simulink model "fig82_SistemaFiltroSintonizado"  (R2021a)
settings: Solver=VariableStepAuto  StartTime=0.0  StopTime=5/60  FixedStep=1/(60*512)  MaxStep=0.1e-3  RelTol=1e-3  EnableMultiTasking=on
InitFcn:
  | Ts = 1/(60*512);
undefined symbols (not defined in the file): D11, Delta
libraries: spsCurrentMeasurementLib x27, spsVoltageMeasurementLib x23, spsSeriesRLCBranchLib x7, spsFourierLib x6, spsThreePhaseTransformerTwoWindingsLib x4, spsUniversalBridgeLib x3, spsTHDLib x3, spsParallelRLCBranchLib x2, spsThreePhaseSeriesRLCBranchLib x1, spsGroundLib x1, spsACCurrentSourceLib x1, spsImpedanceMeasurementLib x1
settings Model: Creator=ajust  LastModifiedBy=ajust
settings SolverCC: AlgebraicLoopSolver=TrustRegion
settings DataIOCC: ReturnWorkspaceOutputs=off
settings OptimizationCC: LifeSpan=inf
settings DebuggingCC: AllowSymbolicDim=off  SFUnexpectedBacktrackingDiag=warning  SFNoUnconditionalDefaultTransitionDiag=warning  SFExecutionAtInitializationDiag=none  SFMachineParentedDataDiag=warning  ArithmeticOperatorsInVariantConditions=warning
settings ModelReferenceCC: PropagateSignalLabelsOutOfModel=off
settings SFSimCC: SimUseLocalCustomCode=off  CustomCodeUndefinedFunction=UseInterfaceOnly
settings RTWCC: RTWUseLocalCustomCode=off
settings CodeAppCC: StateflowObjectComments=on
settings GRTTargetCC: TargetLangStandard=C89/C90 (ANSI)
settings ConfigComp: CovMetricSettings=dw  CovSaveCumulativeToWorkspaceVar=on  CovSaveSingleToWorkspaceVar=on  CovExternalEMLEnable=off
settings SimscapeCC: SimscapeNormalizeSystem=off

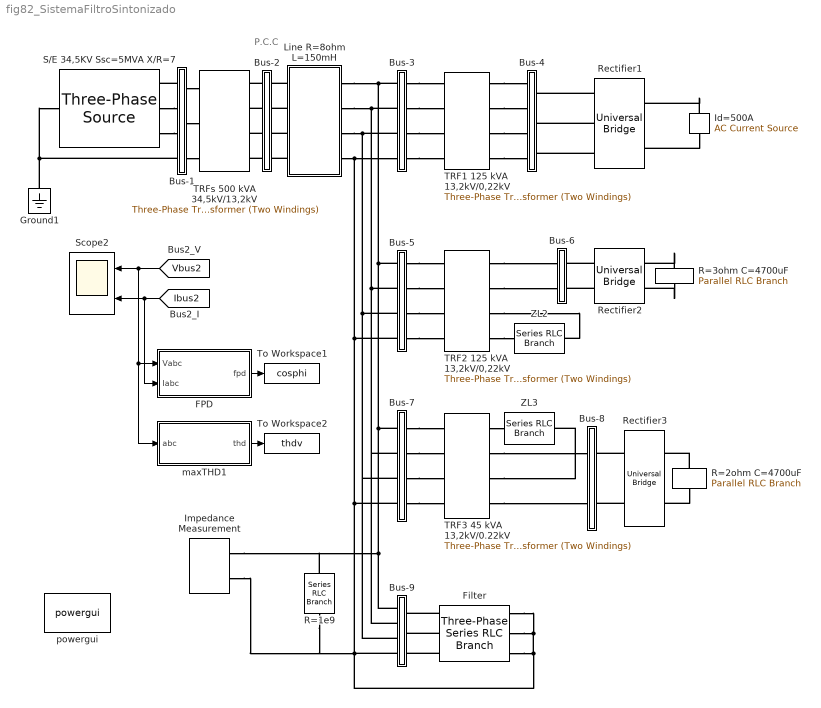
== system fig82_SistemaFiltroSintonizado ==
  note: P.C.C
  Bus-1 : Subsystem
  Bus-2 : Subsystem
  Bus-3 : Subsystem
  Bus-4 : Subsystem
  Bus-5 : Subsystem
  Bus-6 : Subsystem
  Bus-7 : Subsystem
  Bus-8 : Subsystem
  Bus-9 : Subsystem
  FPD : Subsystem
      mask Display:
      | color('blue')
      | disp('Mínimo\nCos(phi)')
  Filter : spsThreePhaseSeriesRLCBranchLib/Three-Phase Series RLC Branch  LConnTagsString=A|B|C  RConnTagsString=A|B|C  BranchType=LC  Resistance=1  Inductance=0.41447  Capacitance=1.8863e-06  Measurements=None
  Ground1 : spsGroundLib/Ground  LConnTagsString=a
  Id=500A : spsACCurrentSourceLib/AC Current Source  Amplitude=500  Phase=90  Frequency=0  SampleTime=0  Measurements=None
      settings: SourceProductBaseCode=PS
  Impedance Measurement : spsImpedanceMeasurementLib/Impedance Measurement  LConnTagsString=+|-  Factor=1
      settings: SourceProductBaseCode=PS
  Line R=8ohm L=150mH : Subsystem
  R=1e9 : spsSeriesRLCBranchLib/Series RLC Branch  LConnTagsString=__new0  RConnTagsString=__new0  BranchType=R  Resistance=1e9  Inductance=1e-3  SetiL0=off  InitialCurrent=0  Capacitance=1e-6  Setx0=off  InitialVoltage=0  Measurements=None
  R=2ohm C=4700uF : spsParallelRLCBranchLib/Parallel RLC Branch  LConnTagsString=a  RConnTagsString=__new0  BranchType=RC  Resistance=2  Inductance=1e-3  SetiL0=off  InitialCurrent=0  Capacitance=4700e-6  Setx0=off  InitialVoltage=220/sqrt(3)  Measurements=None
  R=3ohm C=4700uF : spsParallelRLCBranchLib/Parallel RLC Branch  LConnTagsString=a  RConnTagsString=__new0  BranchType=RC  Resistance=3  Inductance=1e-3  SetiL0=off  InitialCurrent=0  Capacitance=4700e-6  Setx0=off  InitialVoltage=220  Measurements=None
  Rectifier1 : spsUniversalBridgeLib/Universal Bridge  Arms=3  SnubberResistance=1e9  SnubberCapacitance=inf  Device=Diodes  Ron=1e-6  Lon=0  ForwardVoltages="[  0  0  ]"  ForwardVoltage=0  GTOparameters=[ 10e-6 , 20e-6 ]  IGBTparameters=[ 1e-6 , 2e-6 ]  Measurements=None  Measurements_2=None  converterType=Rectifier
  Rectifier2 : spsUniversalBridgeLib/Universal Bridge  Arms=2  SnubberResistance=1e5  SnubberCapacitance=inf  Device=Diodes  Ron=1e-3  Lon=0  ForwardVoltages="[  0  0  ]"  ForwardVoltage=0  GTOparameters=[ 10e-6 , 20e-6 ]  IGBTparameters=[ 1e-6 , 2e-6 ]  Measurements=None  Measurements_2=None  converterType=Rectifier
  Rectifier3 : spsUniversalBridgeLib/Universal Bridge  Arms=2  SnubberResistance=1e5  SnubberCapacitance=inf  Device=Diodes  Ron=1e-3  Lon=0  ForwardVoltages="[  0  0  ]"  ForwardVoltage=0  GTOparameters=[ 10e-6 , 20e-6 ]  IGBTparameters=[ 1e-6 , 2e-6 ]  Measurements=None  Measurements_2=None  converterType=Rectifier
  S/E 34,5KV Ssc=5MVA X/R=7 : spsThreePhaseSourceLib/Three-Phase Source  InternalConnection=Yn  VoltagePhases=off  Voltage=34.5e3  PhaseAngle=0  Voltage_phases=[25e3 25e3 25e3]/sqrt(3)  PhaseAngles_phases=[0 -120 +120]  Frequency=60  NonIdealSource=on  SpecifyImpedance=off  Resistance=33.67  Inductance=0.6251  ShortCircuitLevel=5e6  BaseVoltage=34.5e3  XRratio=7  BusType=swing  Pref=10e3  Qref=0  Prefabc=[10e3, 10e3, 10e3]  Qrefabc=[0, 0, 0]  Qmin=-inf  Qmax=inf
  Scope2 : Scope  NumInputPorts=2
  TRF1 125 kVA 13,2kV/0,22kV : spsThreePhaseTransformerTwoWindingsLib/Three-Phase Transformer (Two Windings)  Winding1Connection=Yn  Winding2Connection=Yn  CoreType=Three single-phase transformers  SetSaturation=off  Hysteresis=off  DataFile='hysteresis'  SetInitialFlux=off  Measurements=None  UNITS=pu  NominalPower=[ 125e3 , 60 ]  Winding1=[ 13.2e3 , 0.002 , 0.08 ]  Winding2=[ 0.22e3 , 0.002 , 0.08 ]  Rm=500  Lm=500  L0=0.5  Saturation=[ 0,0 ; 0.0024,1.2 ; 1.0,1.52 ]  InitialFluxes=[ 0.8 , -0.8 , 0.7 ]  BreakLoop=off  DiscreteSolver=Trapezoidal iterative  DataType=off  TransfoNumber=1
  TRF2 125 kVA 13,2kV/0,22kV : spsThreePhaseTransformerTwoWindingsLib/Three-Phase Transformer (Two Windings)  Winding1Connection=Yn  Winding2Connection=Yn  CoreType=Three single-phase transformers  SetSaturation=off  Hysteresis=off  DataFile='hysteresis'  SetInitialFlux=off  Measurements=None  UNITS=pu  NominalPower=[ 125e3 , 60 ]  Winding1=[ 13.2e3 , 0.002 , 0.08 ]  Winding2=[ 0.22e3 , 0.002 , 0.08 ]  Rm=500  Lm=500  L0=0.5  Saturation=[ 0,0 ; 0.0024,1.2 ; 1.0,1.52 ]  InitialFluxes=[ 0.8 , -0.8 , 0.7 ]  BreakLoop=off  DiscreteSolver=Trapezoidal iterative  DataType=off  TransfoNumber=1
  TRF3 45 kVA 13,2kV/0.22kV : spsThreePhaseTransformerTwoWindingsLib/Three-Phase Transformer (Two Windings)  Winding1Connection=Yn  Winding2Connection=Yn  CoreType=Three single-phase transformers  SetSaturation=off  Hysteresis=off  DataFile='hysteresis'  SetInitialFlux=off  Measurements=None  UNITS=pu  NominalPower=[ 45e3 , 60 ]  Winding1=[ 13.2e3 , 0.002 , 0.08 ]  Winding2=[ 0.22e3 , 0.002 , 0.08 ]  Rm=500  Lm=500  L0=0.5  Saturation=[ 0,0 ; 0.0024,1.2 ; 1.0,1.52 ]  InitialFluxes=[ 0.8 , -0.8 , 0.7 ]  BreakLoop=off  DiscreteSolver=Trapezoidal iterative  DataType=off  TransfoNumber=1
  TRFs 500 kVA 34,5kV/13,2kV : spsThreePhaseTransformerTwoWindingsLib/Three-Phase Transformer (Two Windings)  Winding1Connection=Delta (D11)  Winding2Connection=Yn  CoreType=Three single-phase transformers  SetSaturation=off  Hysteresis=off  DataFile='hysteresis'  SetInitialFlux=off  Measurements=None  UNITS=pu  NominalPower=[ 500e3 , 60 ]  Winding1=[34500 0.002 0.08]  Winding2=[13200 0.002 0.08]  Rm=500.01  Lm=500  L0=9.4717  Saturation=[0 0;0.0024 1.2;0.99999 1.52]  InitialFluxes=[103.54 -103.54 90.594]  BreakLoop=off  DiscreteSolver=Trapezoidal iterative  DataType=off  TransfoNumber=1
  To Workspace1 : ToWorkspace  VariableName=cosphi  SampleTime=-1
  To Workspace2 : ToWorkspace  VariableName=thdv  SampleTime=-1
  ZL2 : spsSeriesRLCBranchLib/Series RLC Branch  LConnTagsString=__new0  RConnTagsString=__new0  BranchType=RL  Resistance=0.1304  Inductance=0.2593/(2*pi*60)  SetiL0=off  InitialCurrent=0  Capacitance=1e-6  Setx0=off  InitialVoltage=0  Measurements=None
  ZL3 : spsSeriesRLCBranchLib/Series RLC Branch  LConnTagsString=__new0  RConnTagsString=__new0  BranchType=RL  Resistance=0.8902  Inductance=1.4641/(2*pi*60)  SetiL0=off  InitialCurrent=0  Capacitance=1e-6  Setx0=off  InitialVoltage=0  Measurements=None
  maxTHD1 : Subsystem
      mask Display:
      | color('blue')
      | disp('Máximo\nTHD')
  powergui : spspowerguiLib/powergui  Priority=1  SimulationMode=Discrete  SampleTime=Ts  frequency=60  Iterations=50  frequencyindice=60  Pbase=100e6  ErrMax=1e-4  UnitsV=kV  UnitsW=MW  buscounter=0  FunctionMessages=off  echomessages=off  EnableUseOfTLC=off  CurrentSourceSwitches=off  DisableSnubberDevices=off  DisableRonSwitches=off  DisableVfSwitches=off  DisplayEquations=off  AutomaticDiscreteSolvers=off  SolverType=Tustin/Backward Euler (TBE)  Interpol=off  ExternalGateDelay=off  methode=off  Ts=10  x0status=blocks  SPID=off  SwTol=0  HookPort=off  NonlinearTolerance=1e-4  nMaxIteration=100  ContinueOnMaxIteration=off  RestoreLinks=warning  ResistiveCurrentMeasurement=off  Frange=[0:2:1000]  Ylog=off  Xlog=off  ShowGrid=on  save=on  variable=ZData  structure=ScopeData  ZoomFFT=off  StartTime=5/60  cycles=1  DisplayStyle=2  fundamental=60  FreqAxis=on  MaxFrequency=1200  frequencyindicesteady=1  RmsSteady=2  display=off
  wires:
  [Vbus2] -> maxTHD1/1(abc), FPD/1(Vabc), Scope2/1
  FPD/1(fpd) -> To Workspace1/1
  [Ibus2] -> FPD/2(Iabc), Scope2/2
  maxTHD1/1(thd) -> To Workspace2/1
  connections:
  Rectifier2/LConn2 -- Bus-6/RConn2
  Bus-3/LConn1 -- Bus-5/LConn1 -- R=1e9/LConn1 -- Impedance Measurement/LConn1 -- Bus-9/LConn1 -- Bus-7/LConn1 -- Line R=8ohm L=150mH/RConn1
  Bus-3/LConn2 -- Bus-5/LConn2 -- Bus-9/LConn2 -- Bus-7/LConn2 -- Line R=8ohm L=150mH/RConn2
  Bus-3/LConn3 -- Bus-5/LConn3 -- Bus-9/LConn3 -- Bus-7/LConn3 -- Line R=8ohm L=150mH/RConn3
  Bus-2/LConn1 -- TRFs 500 kVA 34,5kV/13,2kV/RConn1
  Bus-2/LConn2 -- TRFs 500 kVA 34,5kV/13,2kV/RConn2
  Bus-2/LConn3 -- TRFs 500 kVA 34,5kV/13,2kV/RConn3
  Bus-2/LConn4 -- TRFs 500 kVA 34,5kV/13,2kV/RConn4
  Bus-1/LConn1 -- S/E 34,5KV Ssc=5MVA X/R=7/RConn1
  S/E 34,5KV Ssc=5MVA X/R=7/RConn2 -- Bus-1/LConn2
  S/E 34,5KV Ssc=5MVA X/R=7/RConn3 -- Bus-1/LConn3
  Bus-1/RConn1 -- TRFs 500 kVA 34,5kV/13,2kV/LConn1
  Bus-1/RConn2 -- TRFs 500 kVA 34,5kV/13,2kV/LConn2
  Bus-1/RConn3 -- TRFs 500 kVA 34,5kV/13,2kV/LConn3
  Filter/LConn1 -- Bus-9/RConn1
  Filter/LConn2 -- Bus-9/RConn2
  Filter/LConn3 -- Bus-9/RConn3
  Bus-3/RConn4 -- TRF1 125 kVA 13,2kV/0,22kV/LConn4
  Bus-3/RConn1 -- TRF1 125 kVA 13,2kV/0,22kV/LConn1
  Bus-3/RConn2 -- TRF1 125 kVA 13,2kV/0,22kV/LConn2
  Bus-3/RConn3 -- TRF1 125 kVA 13,2kV/0,22kV/LConn3
  Rectifier1/LConn1 -- Bus-4/RConn1
  Rectifier1/LConn2 -- Bus-4/RConn2
  Rectifier1/LConn3 -- Bus-4/RConn3
  Bus-1/LConn4 -- S/E 34,5KV Ssc=5MVA X/R=7/LConn1 -- Ground1/LConn1
  TRF1 125 kVA 13,2kV/0,22kV/RConn1 -- Bus-4/LConn1
  TRF1 125 kVA 13,2kV/0,22kV/RConn2 -- Bus-4/LConn2
  TRF1 125 kVA 13,2kV/0,22kV/RConn3 -- Bus-4/LConn3
  TRF1 125 kVA 13,2kV/0,22kV/RConn4 -- Bus-4/LConn4
  Line R=8ohm L=150mH/LConn1 -- Bus-2/RConn1
  Line R=8ohm L=150mH/LConn2 -- Bus-2/RConn2
  Line R=8ohm L=150mH/LConn3 -- Bus-2/RConn3
  Line R=8ohm L=150mH/LConn4 -- Bus-2/RConn4
  Rectifier2/LConn1 -- Bus-6/RConn1
  TRF2 125 kVA 13,2kV/0,22kV/RConn1 -- Bus-6/LConn1
  Rectifier3/LConn2 -- Bus-8/RConn2
  Rectifier3/LConn1 -- Bus-8/RConn1
  TRF3 45 kVA 13,2kV/0.22kV/RConn2 -- Bus-8/LConn1
  TRF3 45 kVA 13,2kV/0.22kV/RConn4 -- Bus-8/LConn2
  TRF2 125 kVA 13,2kV/0,22kV/RConn4 -- ZL2/RConn1
  TRF3 45 kVA 13,2kV/0.22kV/RConn3 -- ZL3/RConn1
  TRF3 45 kVA 13,2kV/0.22kV/RConn1 -- ZL3/LConn1
  Bus-5/RConn1 -- TRF2 125 kVA 13,2kV/0,22kV/LConn1
  Bus-5/RConn2 -- TRF2 125 kVA 13,2kV/0,22kV/LConn2
  Bus-5/RConn3 -- TRF2 125 kVA 13,2kV/0,22kV/LConn3
  Bus-5/RConn4 -- TRF2 125 kVA 13,2kV/0,22kV/LConn4
  TRF2 125 kVA 13,2kV/0,22kV/RConn3 -- ZL2/LConn1
  TRF2 125 kVA 13,2kV/0,22kV/RConn2 -- Bus-6/LConn2
  Id=500A/RConn1 -- Rectifier1/RConn2
  Id=500A/LConn1 -- Rectifier1/RConn1
  R=3ohm C=4700uF/RConn1 -- Rectifier2/RConn2
  R=3ohm C=4700uF/LConn1 -- Rectifier2/RConn1
  R=2ohm C=4700uF/LConn1 -- Rectifier3/RConn1
  R=2ohm C=4700uF/RConn1 -- Rectifier3/RConn2
  Bus-7/RConn1 -- TRF3 45 kVA 13,2kV/0.22kV/LConn1
  Bus-7/RConn2 -- TRF3 45 kVA 13,2kV/0.22kV/LConn2
  Bus-7/RConn3 -- TRF3 45 kVA 13,2kV/0.22kV/LConn3
  Bus-7/RConn4 -- TRF3 45 kVA 13,2kV/0.22kV/LConn4
  Filter/RConn3 -- Bus-9/LConn4 -- R=1e9/RConn1 -- Impedance Measurement/LConn2 -- Bus-7/LConn4 -- Bus-5/LConn4 -- Line R=8ohm L=150mH/RConn4 -- Bus-3/LConn4 -- Filter/RConn2 -- Filter/RConn1

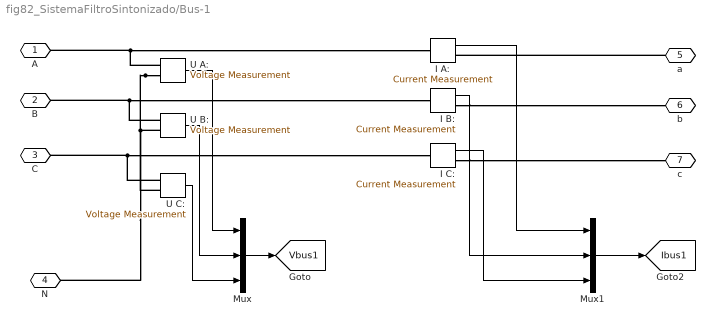
== system fig82_SistemaFiltroSintonizado/Bus-1 ==
  I A: : spsCurrentMeasurementLib/Current Measurement  PhasorSimulation=off  OutputType=Complex  PSBequivalent=0
  I B: : spsCurrentMeasurementLib/Current Measurement  PhasorSimulation=off  OutputType=Complex  PSBequivalent=0
  I C: : spsCurrentMeasurementLib/Current Measurement  PhasorSimulation=off  OutputType=Complex  PSBequivalent=0
  Mux : Mux  Inputs=3
  Mux1 : Mux  Inputs=3
  U A: : spsVoltageMeasurementLib/Voltage Measurement  PhasorSimulation=off  OutputType=Complex  PSBequivalent=0
  U B: : spsVoltageMeasurementLib/Voltage Measurement  PhasorSimulation=off  OutputType=Complex  PSBequivalent=0
  U C: : spsVoltageMeasurementLib/Voltage Measurement  PhasorSimulation=off  OutputType=Complex  PSBequivalent=0
  A : PMIOPort  Side=Left
  B : PMIOPort  Port=2  Side=Left
  C : PMIOPort  Port=3  Side=Left
  N : PMIOPort  Port=4  Side=Left
  a : PMIOPort  Port=5  Side=Right
  b : PMIOPort  Port=6  Side=Right
  c : PMIOPort  Port=7  Side=Right
  tag scope: Ibus1=global, Vbus1=global
  wires:
  U A:/1 -> Mux/1
  U B:/1 -> Mux/2
  Mux1/1 -> [Ibus1]
  Mux/1 -> [Vbus1]
  I C:/1 -> Mux1/3
  U C:/1 -> Mux/3
  I B:/1 -> Mux1/2
  I A:/1 -> Mux1/1
  connections:
  U A:/LConn1 -- I A:/LConn1 -- A/RConn1
  U B:/LConn1 -- I B:/LConn1 -- B/RConn1
  U A:/LConn2 -- U B:/LConn2 -- U C:/LConn2 -- N/RConn1
  U C:/LConn1 -- I C:/LConn1 -- C/RConn1
  I C:/RConn1 -- c/RConn1
  a/RConn1 -- I A:/RConn1
  I B:/RConn1 -- b/RConn1

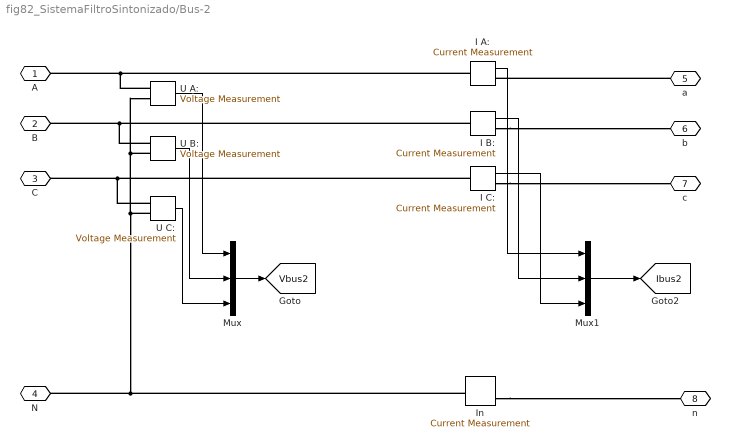
== system fig82_SistemaFiltroSintonizado/Bus-2 ==
  I A: : spsCurrentMeasurementLib/Current Measurement  PhasorSimulation=off  OutputType=Complex  PSBequivalent=0
  I B: : spsCurrentMeasurementLib/Current Measurement  PhasorSimulation=off  OutputType=Complex  PSBequivalent=0
  I C: : spsCurrentMeasurementLib/Current Measurement  PhasorSimulation=off  OutputType=Complex  PSBequivalent=0
  In : spsCurrentMeasurementLib/Current Measurement  PhasorSimulation=off  OutputType=Complex  PSBequivalent=0
  Mux : Mux  Inputs=3
  Mux1 : Mux  Inputs=3
  U A: : spsVoltageMeasurementLib/Voltage Measurement  PhasorSimulation=off  OutputType=Complex  PSBequivalent=0
  U B: : spsVoltageMeasurementLib/Voltage Measurement  PhasorSimulation=off  OutputType=Complex  PSBequivalent=0
  U C: : spsVoltageMeasurementLib/Voltage Measurement  PhasorSimulation=off  OutputType=Complex  PSBequivalent=0
  A : PMIOPort  Side=Left
  B : PMIOPort  Port=2  Side=Left
  C : PMIOPort  Port=3  Side=Left
  N : PMIOPort  Port=4  Side=Left
  a : PMIOPort  Port=5  Side=Right
  b : PMIOPort  Port=6  Side=Right
  c : PMIOPort  Port=7  Side=Right
  n : PMIOPort  Port=8  Side=Right
  tag scope: Ibus2=global, Vbus2=global
  wires:
  U A:/1 -> Mux/1
  U B:/1 -> Mux/2
  Mux1/1 -> [Ibus2]
  Mux/1 -> [Vbus2]
  I C:/1 -> Mux1/3
  U C:/1 -> Mux/3
  I B:/1 -> Mux1/2
  I A:/1 -> Mux1/1
  connections:
  U C:/LConn2 -- N/RConn1 -- In/LConn1 -- U A:/LConn2 -- U B:/LConn2
  In/RConn1 -- n/RConn1
  I A:/LConn1 -- U A:/LConn1 -- A/RConn1
  I B:/LConn1 -- U B:/LConn1 -- B/RConn1
  I C:/LConn1 -- U C:/LConn1 -- C/RConn1
  I C:/RConn1 -- c/RConn1
  a/RConn1 -- I A:/RConn1
  I B:/RConn1 -- b/RConn1

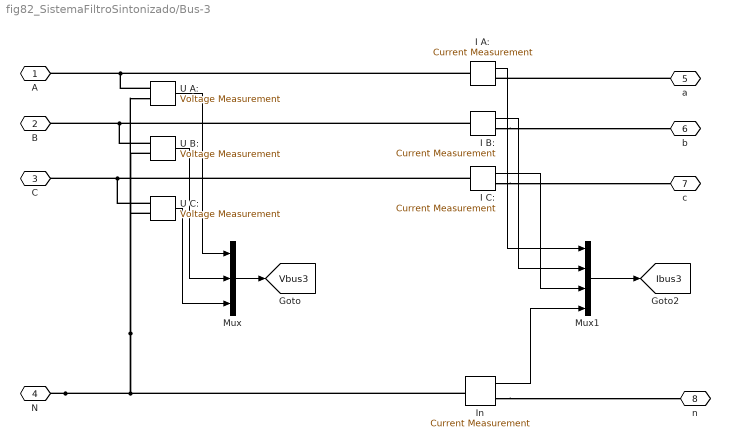
== system fig82_SistemaFiltroSintonizado/Bus-3 ==
  I A: : spsCurrentMeasurementLib/Current Measurement  PhasorSimulation=off  OutputType=Complex  PSBequivalent=0
  I B: : spsCurrentMeasurementLib/Current Measurement  PhasorSimulation=off  OutputType=Complex  PSBequivalent=0
  I C: : spsCurrentMeasurementLib/Current Measurement  PhasorSimulation=off  OutputType=Complex  PSBequivalent=0
  In : spsCurrentMeasurementLib/Current Measurement  PhasorSimulation=off  OutputType=Complex  PSBequivalent=0
  Mux : Mux  Inputs=3
  Mux1 : Mux
  U A: : spsVoltageMeasurementLib/Voltage Measurement  PhasorSimulation=off  OutputType=Complex  PSBequivalent=0
  U B: : spsVoltageMeasurementLib/Voltage Measurement  PhasorSimulation=off  OutputType=Complex  PSBequivalent=0
  U C: : spsVoltageMeasurementLib/Voltage Measurement  PhasorSimulation=off  OutputType=Complex  PSBequivalent=0
  A : PMIOPort  Side=Left
  B : PMIOPort  Port=2  Side=Left
  C : PMIOPort  Port=3  Side=Left
  N : PMIOPort  Port=4  Side=Left
  a : PMIOPort  Port=5  Side=Right
  b : PMIOPort  Port=6  Side=Right
  c : PMIOPort  Port=7  Side=Right
  n : PMIOPort  Port=8  Side=Right
  tag scope: Ibus3=global, Vbus3=global
  wires:
  U A:/1 -> Mux/1
  U B:/1 -> Mux/2
  Mux1/1 -> [Ibus3]
  Mux/1 -> [Vbus3]
  I C:/1 -> Mux1/3
  U C:/1 -> Mux/3
  I B:/1 -> Mux1/2
  I A:/1 -> Mux1/1
  In/1 -> Mux1/4
  connections:
  N/RConn1 -- In/LConn1 -- U A:/LConn2 -- U B:/LConn2 -- U C:/LConn2
  In/RConn1 -- n/RConn1
  I A:/LConn1 -- A/RConn1 -- U A:/LConn1
  I B:/LConn1 -- B/RConn1 -- U B:/LConn1
  I C:/LConn1 -- C/RConn1 -- U C:/LConn1
  I C:/RConn1 -- c/RConn1
  a/RConn1 -- I A:/RConn1
  I B:/RConn1 -- b/RConn1

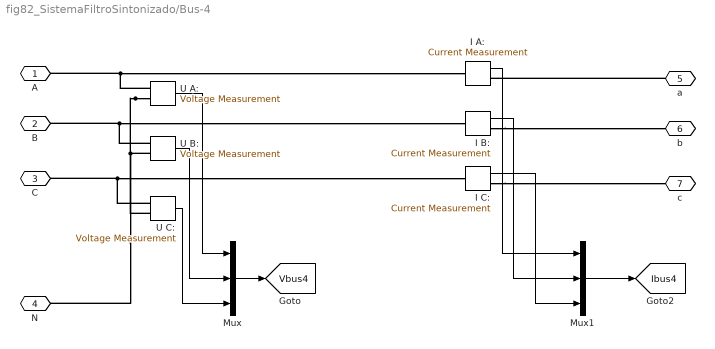
== system fig82_SistemaFiltroSintonizado/Bus-4 ==
  I A: : spsCurrentMeasurementLib/Current Measurement  PhasorSimulation=off  OutputType=Complex  PSBequivalent=0
  I B: : spsCurrentMeasurementLib/Current Measurement  PhasorSimulation=off  OutputType=Complex  PSBequivalent=0
  I C: : spsCurrentMeasurementLib/Current Measurement  PhasorSimulation=off  OutputType=Complex  PSBequivalent=0
  Mux : Mux  Inputs=3
  Mux1 : Mux  Inputs=3
  U A: : spsVoltageMeasurementLib/Voltage Measurement  PhasorSimulation=off  OutputType=Complex  PSBequivalent=0
  U B: : spsVoltageMeasurementLib/Voltage Measurement  PhasorSimulation=off  OutputType=Complex  PSBequivalent=0
  U C: : spsVoltageMeasurementLib/Voltage Measurement  PhasorSimulation=off  OutputType=Complex  PSBequivalent=0
  A : PMIOPort  Side=Left
  B : PMIOPort  Port=2  Side=Left
  C : PMIOPort  Port=3  Side=Left
  N : PMIOPort  Port=4  Side=Left
  a : PMIOPort  Port=5  Side=Right
  b : PMIOPort  Port=6  Side=Right
  c : PMIOPort  Port=7  Side=Right
  tag scope: Ibus4=global, Vbus4=global
  wires:
  U A:/1 -> Mux/1
  U B:/1 -> Mux/2
  Mux1/1 -> [Ibus4]
  Mux/1 -> [Vbus4]
  I C:/1 -> Mux1/3
  U C:/1 -> Mux/3
  I B:/1 -> Mux1/2
  I A:/1 -> Mux1/1
  connections:
  U A:/LConn1 -- A/RConn1 -- I A:/LConn1
  U B:/LConn1 -- B/RConn1 -- I B:/LConn1
  U A:/LConn2 -- U B:/LConn2 -- U C:/LConn2 -- N/RConn1
  U C:/LConn1 -- C/RConn1 -- I C:/LConn1
  I C:/RConn1 -- c/RConn1
  a/RConn1 -- I A:/RConn1
  I B:/RConn1 -- b/RConn1

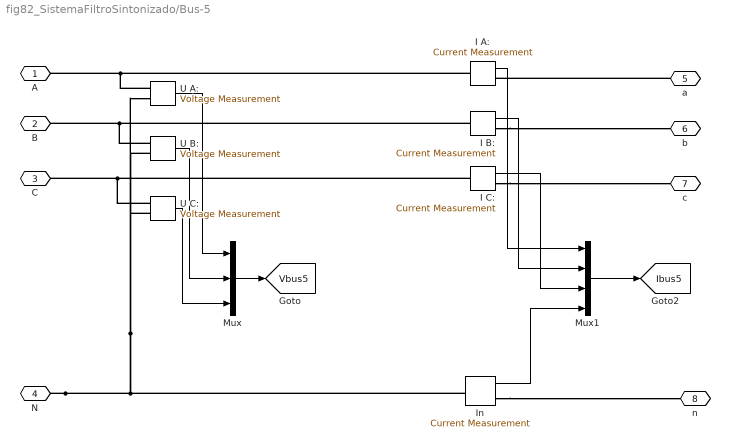
== system fig82_SistemaFiltroSintonizado/Bus-5 ==
  I A: : spsCurrentMeasurementLib/Current Measurement  PhasorSimulation=off  OutputType=Complex  PSBequivalent=0
  I B: : spsCurrentMeasurementLib/Current Measurement  PhasorSimulation=off  OutputType=Complex  PSBequivalent=0
  I C: : spsCurrentMeasurementLib/Current Measurement  PhasorSimulation=off  OutputType=Complex  PSBequivalent=0
  In : spsCurrentMeasurementLib/Current Measurement  PhasorSimulation=off  OutputType=Complex  PSBequivalent=0
  Mux : Mux  Inputs=3
  Mux1 : Mux
  U A: : spsVoltageMeasurementLib/Voltage Measurement  PhasorSimulation=off  OutputType=Complex  PSBequivalent=0
  U B: : spsVoltageMeasurementLib/Voltage Measurement  PhasorSimulation=off  OutputType=Complex  PSBequivalent=0
  U C: : spsVoltageMeasurementLib/Voltage Measurement  PhasorSimulation=off  OutputType=Complex  PSBequivalent=0
  A : PMIOPort  Side=Left
  B : PMIOPort  Port=2  Side=Left
  C : PMIOPort  Port=3  Side=Left
  N : PMIOPort  Port=4  Side=Left
  a : PMIOPort  Port=5  Side=Right
  b : PMIOPort  Port=6  Side=Right
  c : PMIOPort  Port=7  Side=Right
  n : PMIOPort  Port=8  Side=Right
  tag scope: Ibus5=global, Vbus5=global
  wires:
  U A:/1 -> Mux/1
  U B:/1 -> Mux/2
  Mux1/1 -> [Ibus5]
  Mux/1 -> [Vbus5]
  I C:/1 -> Mux1/3
  U C:/1 -> Mux/3
  I B:/1 -> Mux1/2
  I A:/1 -> Mux1/1
  In/1 -> Mux1/4
  connections:
  N/RConn1 -- In/LConn1 -- U A:/LConn2 -- U B:/LConn2 -- U C:/LConn2
  In/RConn1 -- n/RConn1
  I A:/LConn1 -- A/RConn1 -- U A:/LConn1
  I B:/LConn1 -- B/RConn1 -- U B:/LConn1
  I C:/LConn1 -- C/RConn1 -- U C:/LConn1
  I C:/RConn1 -- c/RConn1
  a/RConn1 -- I A:/RConn1
  I B:/RConn1 -- b/RConn1

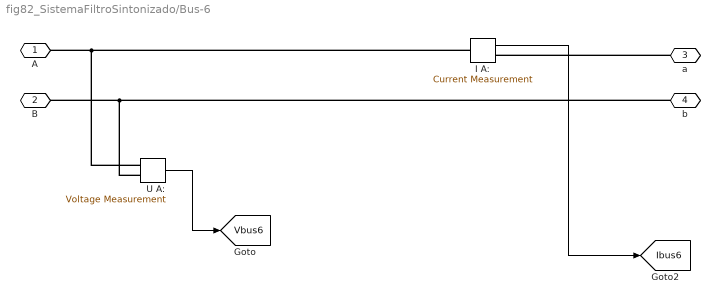
== system fig82_SistemaFiltroSintonizado/Bus-6 ==
  I A: : spsCurrentMeasurementLib/Current Measurement  PhasorSimulation=off  OutputType=Complex  PSBequivalent=0
  U A: : spsVoltageMeasurementLib/Voltage Measurement  PhasorSimulation=off  OutputType=Complex  PSBequivalent=0
  A : PMIOPort  Side=Left
  B : PMIOPort  Port=2  Side=Left
  a : PMIOPort  Port=3  Side=Right
  b : PMIOPort  Port=4  Side=Right
  tag scope: Ibus6=global, Vbus6=global
  wires:
  U A:/1 -> [Vbus6]
  I A:/1 -> [Ibus6]
  connections:
  I A:/LConn1 -- A/RConn1 -- U A:/LConn1
  U A:/LConn2 -- b/RConn1 -- B/RConn1
  a/RConn1 -- I A:/RConn1

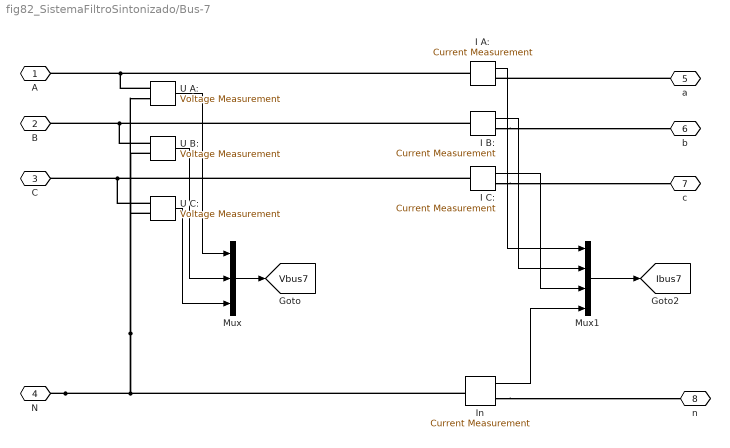
== system fig82_SistemaFiltroSintonizado/Bus-7 ==
  I A: : spsCurrentMeasurementLib/Current Measurement  PhasorSimulation=off  OutputType=Complex  PSBequivalent=0
  I B: : spsCurrentMeasurementLib/Current Measurement  PhasorSimulation=off  OutputType=Complex  PSBequivalent=0
  I C: : spsCurrentMeasurementLib/Current Measurement  PhasorSimulation=off  OutputType=Complex  PSBequivalent=0
  In : spsCurrentMeasurementLib/Current Measurement  PhasorSimulation=off  OutputType=Complex  PSBequivalent=0
  Mux : Mux  Inputs=3
  Mux1 : Mux
  U A: : spsVoltageMeasurementLib/Voltage Measurement  PhasorSimulation=off  OutputType=Complex  PSBequivalent=0
  U B: : spsVoltageMeasurementLib/Voltage Measurement  PhasorSimulation=off  OutputType=Complex  PSBequivalent=0
  U C: : spsVoltageMeasurementLib/Voltage Measurement  PhasorSimulation=off  OutputType=Complex  PSBequivalent=0
  A : PMIOPort  Side=Left
  B : PMIOPort  Port=2  Side=Left
  C : PMIOPort  Port=3  Side=Left
  N : PMIOPort  Port=4  Side=Left
  a : PMIOPort  Port=5  Side=Right
  b : PMIOPort  Port=6  Side=Right
  c : PMIOPort  Port=7  Side=Right
  n : PMIOPort  Port=8  Side=Right
  tag scope: Ibus7=global, Vbus7=global
  wires:
  U A:/1 -> Mux/1
  U B:/1 -> Mux/2
  Mux1/1 -> [Ibus7]
  Mux/1 -> [Vbus7]
  I C:/1 -> Mux1/3
  U C:/1 -> Mux/3
  I B:/1 -> Mux1/2
  I A:/1 -> Mux1/1
  In/1 -> Mux1/4
  connections:
  N/RConn1 -- In/LConn1 -- U A:/LConn2 -- U B:/LConn2 -- U C:/LConn2
  In/RConn1 -- n/RConn1
  I A:/LConn1 -- A/RConn1 -- U A:/LConn1
  I B:/LConn1 -- B/RConn1 -- U B:/LConn1
  I C:/LConn1 -- C/RConn1 -- U C:/LConn1
  I C:/RConn1 -- c/RConn1
  a/RConn1 -- I A:/RConn1
  I B:/RConn1 -- b/RConn1

== system fig82_SistemaFiltroSintonizado/Bus-8 ==
  I A: : spsCurrentMeasurementLib/Current Measurement  PhasorSimulation=off  OutputType=Complex  PSBequivalent=0
  U A: : spsVoltageMeasurementLib/Voltage Measurement  PhasorSimulation=off  OutputType=Complex  PSBequivalent=0
  A : PMIOPort  Side=Left
  B : PMIOPort  Port=2  Side=Left
  a : PMIOPort  Port=3  Side=Right
  b : PMIOPort  Port=4  Side=Right
  tag scope: Ibus8=global, Vbus8=global
  wires:
  U A:/1 -> [Vbus8]
  I A:/1 -> [Ibus8]
  connections:
  I A:/LConn1 -- A/RConn1 -- U A:/LConn1
  a/RConn1 -- I A:/RConn1
  U A:/LConn2 -- B/RConn1 -- b/RConn1

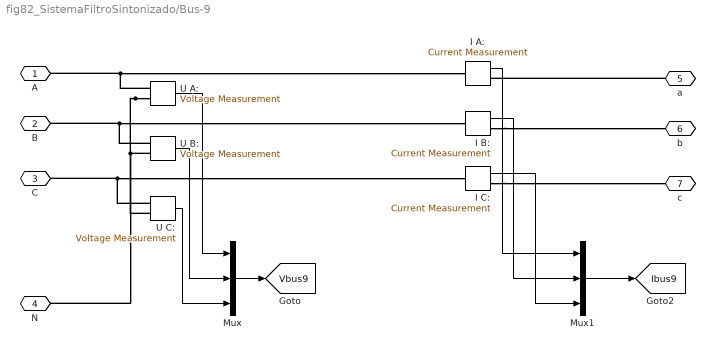
== system fig82_SistemaFiltroSintonizado/Bus-9 ==
  I A: : spsCurrentMeasurementLib/Current Measurement  PhasorSimulation=off  OutputType=Complex  PSBequivalent=0
  I B: : spsCurrentMeasurementLib/Current Measurement  PhasorSimulation=off  OutputType=Complex  PSBequivalent=0
  I C: : spsCurrentMeasurementLib/Current Measurement  PhasorSimulation=off  OutputType=Complex  PSBequivalent=0
  Mux : Mux  Inputs=3
  Mux1 : Mux  Inputs=3
  U A: : spsVoltageMeasurementLib/Voltage Measurement  PhasorSimulation=off  OutputType=Complex  PSBequivalent=0
  U B: : spsVoltageMeasurementLib/Voltage Measurement  PhasorSimulation=off  OutputType=Complex  PSBequivalent=0
  U C: : spsVoltageMeasurementLib/Voltage Measurement  PhasorSimulation=off  OutputType=Complex  PSBequivalent=0
  A : PMIOPort  Side=Left
  B : PMIOPort  Port=2  Side=Left
  C : PMIOPort  Port=3  Side=Left
  N : PMIOPort  Port=4  Side=Left
  a : PMIOPort  Port=5  Side=Right
  b : PMIOPort  Port=6  Side=Right
  c : PMIOPort  Port=7  Side=Right
  tag scope: Ibus9=global, Vbus9=global
  wires:
  U A:/1 -> Mux/1
  U B:/1 -> Mux/2
  Mux1/1 -> [Ibus9]
  Mux/1 -> [Vbus9]
  I C:/1 -> Mux1/3
  U C:/1 -> Mux/3
  I B:/1 -> Mux1/2
  I A:/1 -> Mux1/1
  connections:
  U A:/LConn1 -- A/RConn1 -- I A:/LConn1
  U B:/LConn1 -- B/RConn1 -- I B:/LConn1
  U A:/LConn2 -- U B:/LConn2 -- U C:/LConn2 -- N/RConn1
  U C:/LConn1 -- C/RConn1 -- I C:/LConn1
  I C:/RConn1 -- c/RConn1
  a/RConn1 -- I A:/RConn1
  I B:/RConn1 -- b/RConn1

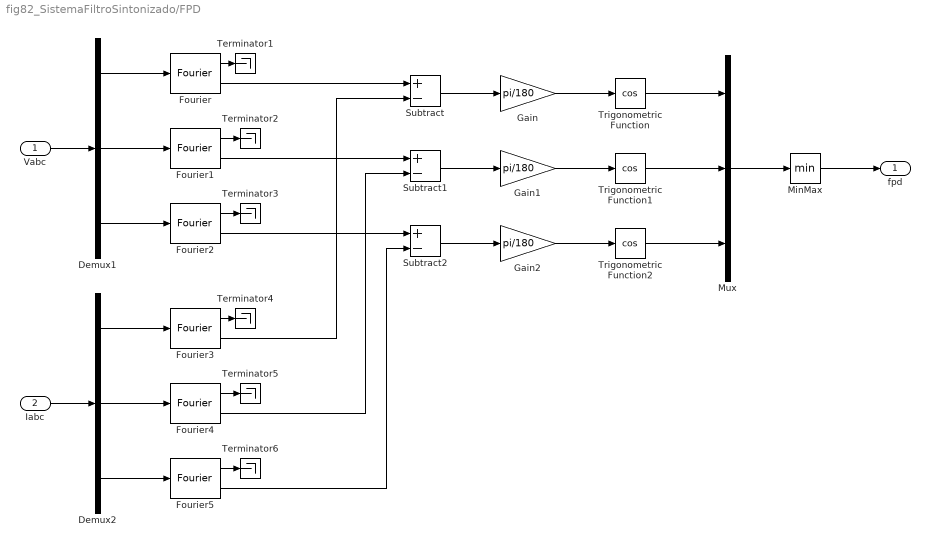
== system fig82_SistemaFiltroSintonizado/FPD ==
  Vabc : Inport
  Iabc : Inport  Port=2
  Demux1 : Demux  Outputs=3
  Demux2 : Demux  Outputs=3
  Fourier{,1..5} (6 alike) : spsFourierLib/Fourier  Freq=60  n=1  InInit=[0, 0]  Ts=0
      settings: SourceProductBaseCode=PS
  Gain : Gain  Gain=pi/180
  Gain1 : Gain  Gain=pi/180
  Gain2 : Gain  Gain=pi/180
  MinMax : MinMax
  Mux : Mux  Inputs=3
  Subtract : Sum  Inputs=+-
  Subtract1 : Sum  Inputs=+-
  Subtract2 : Sum  Inputs=+-
  Terminator{1..6} (6 alike) : Terminator
  Trigonometric Function : Trigonometry  Operator=cos
  Trigonometric Function1 : Trigonometry  Operator=cos
  Trigonometric Function2 : Trigonometry  Operator=cos
  fpd : Outport
  wires:
  Gain2/1 -> Trigonometric Function2/1
  Gain1/1 -> Trigonometric Function1/1
  Gain/1 -> Trigonometric Function/1
  Subtract/1 -> Gain/1
  Fourier5/2 -> Subtract2/2
  Fourier2/2 -> Subtract2/1
  Fourier4/2 -> Subtract1/2
  Fourier1/2 -> Subtract1/1
  Trigonometric Function2/1 -> Mux/3
  Subtract2/1 -> Gain2/1
  Trigonometric Function1/1 -> Mux/2
  Subtract1/1 -> Gain1/1
  Trigonometric Function/1 -> Mux/1
  Mux/1 -> MinMax/1
  MinMax/1 -> fpd/1
  Fourier3/2 -> Subtract/2
  Fourier/2 -> Subtract/1
  Fourier5/1 -> Terminator6/1
  Demux2/2 -> Fourier4/1
  Demux2/3 -> Fourier5/1
  Iabc/1 -> Demux2/1
  Demux2/1 -> Fourier3/1
  Fourier3/1 -> Terminator4/1
  Fourier4/1 -> Terminator5/1
  Fourier2/1 -> Terminator3/1
  Fourier1/1 -> Terminator2/1
  Fourier/1 -> Terminator1/1
  Demux1/3 -> Fourier2/1
  Demux1/2 -> Fourier1/1
  Demux1/1 -> Fourier/1
  Vabc/1 -> Demux1/1

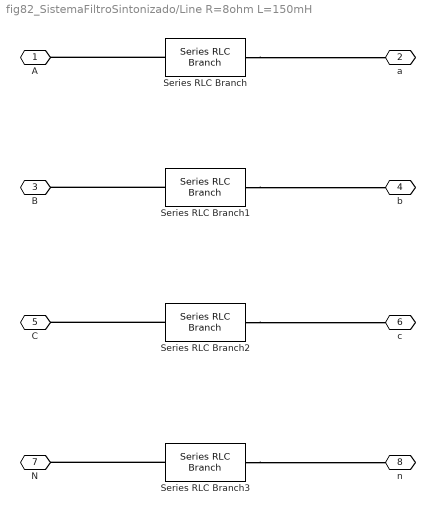
== system fig82_SistemaFiltroSintonizado/Line R=8ohm L=150mH ==
  Series RLC Branch{,1..3} (4 alike) : spsSeriesRLCBranchLib/Series RLC Branch  LConnTagsString=__new0  RConnTagsString=__new0  BranchType=RL  Resistance=8  Inductance=150e-3  SetiL0=off  InitialCurrent=0  Capacitance=1e-6  Setx0=off  InitialVoltage=0  Measurements=None
  A : PMIOPort  Side=Left
  a : PMIOPort  Port=2  Side=Right
  B : PMIOPort  Port=3  Side=Left
  b : PMIOPort  Port=4  Side=Right
  C : PMIOPort  Port=5  Side=Left
  c : PMIOPort  Port=6  Side=Right
  N : PMIOPort  Port=7  Side=Left
  n : PMIOPort  Port=8  Side=Right
  connections:
  Series RLC Branch3/RConn1 -- n/RConn1
  Series RLC Branch3/LConn1 -- N/RConn1
  Series RLC Branch/LConn1 -- A/RConn1
  Series RLC Branch1/LConn1 -- B/RConn1
  Series RLC Branch2/LConn1 -- C/RConn1
  Series RLC Branch/RConn1 -- a/RConn1
  Series RLC Branch2/RConn1 -- c/RConn1
  Series RLC Branch1/RConn1 -- b/RConn1

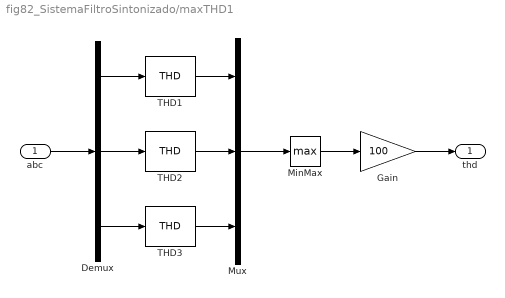
== system fig82_SistemaFiltroSintonizado/maxTHD1 ==
  abc : Inport
  Demux : Demux  Outputs=3
  Gain : Gain  Gain=100
  MinMax : MinMax  Function=max
  Mux : Mux  Inputs=3
  THD1 : spsTHDLib/THD  Freq=60  Ts=0
      settings: SourceProductBaseCode=PS
  THD2 : spsTHDLib/THD  Freq=60  Ts=0
      settings: SourceProductBaseCode=PS
  THD3 : spsTHDLib/THD  Freq=60  Ts=0
      settings: SourceProductBaseCode=PS
  thd : Outport
  wires:
  Gain/1 -> thd/1
  MinMax/1 -> Gain/1
  THD3/1 -> Mux/3
  THD2/1 -> Mux/2
  THD1/1 -> Mux/1
  Mux/1 -> MinMax/1
  Demux/3 -> THD3/1
  Demux/2 -> THD2/1
  Demux/1 -> THD1/1
  abc/1 -> Demux/1
